simulink model "R19_Modelo_control_CORRIENTE_c_2GDL_2021"  (R2019a)
settings: Solver=ode45  StartTime=0.0  StopTime=20  RelTol=1e-9
undefined symbols (not defined in the file): currentSensorNoise, DiscIntNeverNeededParam, dtCurrent, dTSensor, filterConstant, initial_conds, K_c, Ki, Kp, Lcoil, noiseSensor, pod, Rcoil, T, tauFilterCurrent, z_0, z_ini
libraries: simulink x3, shared3dof x1, cstblocks x1, simulink_extras x1
settings Model: Creator=skapa  LastModifiedBy=emate
settings DataIOCC: LimitDataPoints=on  SaveFormat=Array  SignalLoggingSaveFormat=ModelDataLogs  ReturnWorkspaceOutputs=off
settings OptimizationCC: BlockReduction=off  BooleanDataType=off  LifeSpan=inf
settings DebuggingCC: SaveWithParameterizedLinksMsg=none  UnderspecifiedInitializationDetection=Classic  MergeDetectMultiDrivingBlocksExec=none  SignalResolutionControl=TryResolveAllWithWarning  MultiTaskDSMMsg=warning  MultiTaskCondExecSysMsg=none  SFUnexpectedBacktrackingDiag=warning  SFNoUnconditionalDefaultTransitionDiag=warning  SFExecutionAtInitializationDiag=none  ArithmeticOperatorsInVariantConditions=warning
settings HardwareCC: ProdBitPerPointer=32  ProdBitPerSizeT=32  ProdBitPerPtrDiffT=32  ProdLargestAtomicFloat=None  ProdIntDivRoundTo=Undefined  ProdEndianess=Unspecified  ProdWordSize=32  ProdHWDeviceType=32-bit Generic  TargetUnknown=on
settings ModelReferenceCC: PropagateSignalLabelsOutOfModel=off
settings SFSimCC: SimUseLocalCustomCode=off
settings RTWCC: RTWUseLocalCustomCode=off
settings CodeAppCC: StateflowObjectComments=on
settings GRTTargetCC: TargetLangStandard=C89/C90 (ANSI)
settings ConfigComp: CovMetricSettings=dw  CovSaveCumulativeToWorkspaceVar=on  CovSaveSingleToWorkspaceVar=on  CovExternalEMLEnable=off

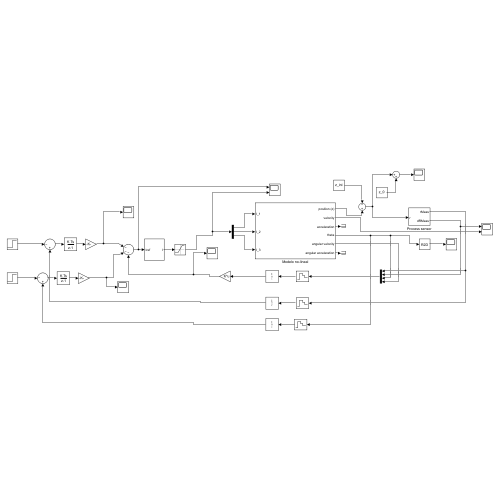
[thumbnail: Simulink's stored preview of the top-level diagram]
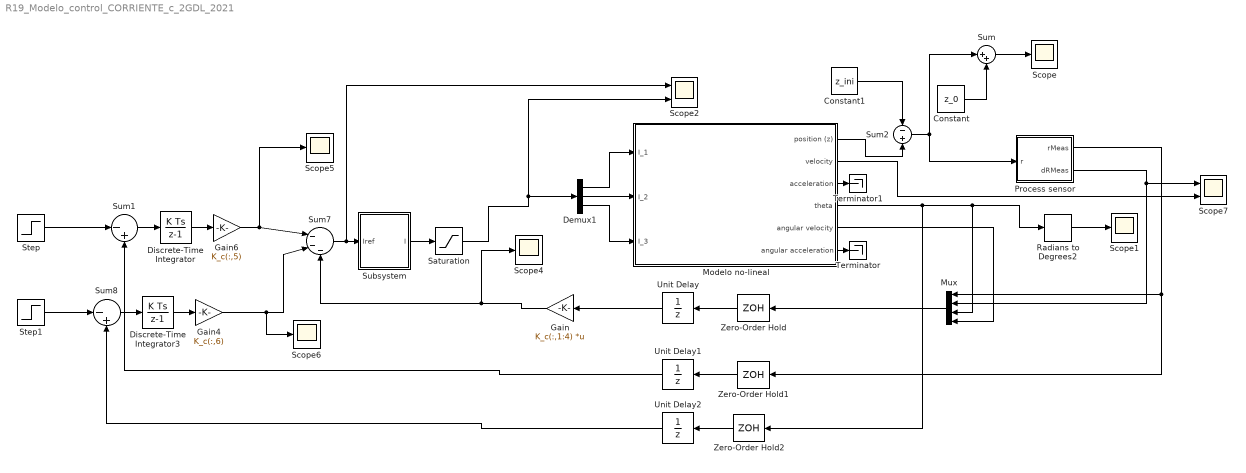
== system R19_Modelo_control_CORRIENTE_c_2GDL_2021 ==
  Constant : Constant  Value=z_0
  Constant1 : Constant  Value=z_ini  SampleTime=T
  Demux1 : Demux  Outputs=3
  Discrete-Time Integrator : DiscreteIntegrator  SampleTime=T  ICPrevOutput=DiscIntNeverNeededParam  ICPrevScaledInput=DiscIntNeverNeededParam
  Discrete-Time Integrator3 : DiscreteIntegrator  SampleTime=T  ICPrevOutput=DiscIntNeverNeededParam  ICPrevScaledInput=DiscIntNeverNeededParam
  Gain : Gain  Gain=K_c(:,1:4)  Multiplication=Matrix(K*u)
  Gain4 : Gain  Gain=K_c(:,6)
  Gain6 : Gain  Gain=K_c(:,5)
  Modelo no-lineal : Subsystem
  Mux : Mux
  Process sensor : Subsystem
  Radians to Degrees2 : simulink_extras/Transformations/Radians to Degrees
  Saturation : Saturate  UpperLimit=40  LowerLimit=-40
  Scope{,1,4..6} (5 alike) : Scope
  Scope2 : Scope  NumInputPorts=2
  Scope7 : Scope  NumInputPorts=2
  Step : Step  Time=0  After=0  SampleTime=T
  Step1 : Step  Time=0  After=0  SampleTime=T
  Subsystem : Subsystem
  Sum : Sum  Inputs=|++
  Sum1 : Sum  Inputs=|-+
  Sum2 : Sum  Inputs=-|+
  Sum7 : Sum  Inputs=|---
  Sum8 : Sum  Inputs=|-+
  Terminator : Terminator
  Terminator1 : Terminator
  Unit Delay : UnitDelay  InitialCondition=[0,0,0,0]  SampleTime=-1  HasFrameUpgradeWarning=on
  Unit Delay1 : UnitDelay  InitialCondition=[0]  SampleTime=-1  HasFrameUpgradeWarning=on
  Unit Delay2 : UnitDelay  InitialCondition=[0]  SampleTime=-1  HasFrameUpgradeWarning=on
  Zero-Order Hold : ZeroOrderHold  SampleTime=T
  Zero-Order Hold1 : ZeroOrderHold  SampleTime=T
  Zero-Order Hold2 : ZeroOrderHold  SampleTime=T
  wires:
  Sum1/1 -> Discrete-Time Integrator/1
  Discrete-Time Integrator/1 -> Gain6/1
  Gain6/1 -> Scope5/1, Sum7/1
  Demux1/1 -> Modelo no-lineal/1(I_1)
  Demux1/2 -> Modelo no-lineal/2(I_2)
  Demux1/3 -> Modelo no-lineal/3(I_3)
  Modelo no-lineal/4(theta) -> Zero-Order Hold2/1, Mux/3, Radians to Degrees2/1
  Modelo no-lineal/6(angular acceleration) -> Terminator/1
  Unit Delay/1 -> Gain/1
  Sum2/1 -> Sum/1, Process sensor/1(r)
  Modelo no-lineal/1(position (z)) -> Sum2/2
  Constant1/1 -> Sum2/1
  Unit Delay1/1 -> Sum1/2
  Step/1 -> Sum1/1
  Gain/1 -> Scope4/1, Sum7/3
  Step1/1 -> Sum8/1
  Discrete-Time Integrator3/1 -> Gain4/1
  Sum8/1 -> Discrete-Time Integrator3/1
  Unit Delay2/1 -> Sum8/2
  Modelo no-lineal/3(acceleration) -> Terminator1/1
  Radians to Degrees2/1 -> Scope1/1
  Saturation/1 -> Scope2/2, Demux1/1
  Zero-Order Hold/1 -> Unit Delay/1
  Zero-Order Hold1/1 -> Unit Delay1/1
  Zero-Order Hold2/1 -> Unit Delay2/1
  Process sensor/1(rMeas) -> Mux/1, Zero-Order Hold1/1
  Modelo no-lineal/5(angular velocity) -> Mux/4
  Mux/1 -> Zero-Order Hold/1
  Process sensor/2(dRMeas) -> Scope7/1, Mux/2
  Modelo no-lineal/2(velocity) -> Scope7/2
  Gain4/1 -> Scope6/1, Sum7/2
  Constant/1 -> Sum/2
  Sum/1 -> Scope/1
  Sum7/1 -> Scope2/1, Subsystem/1(Iref)
  Subsystem/1(I) -> Saturation/1

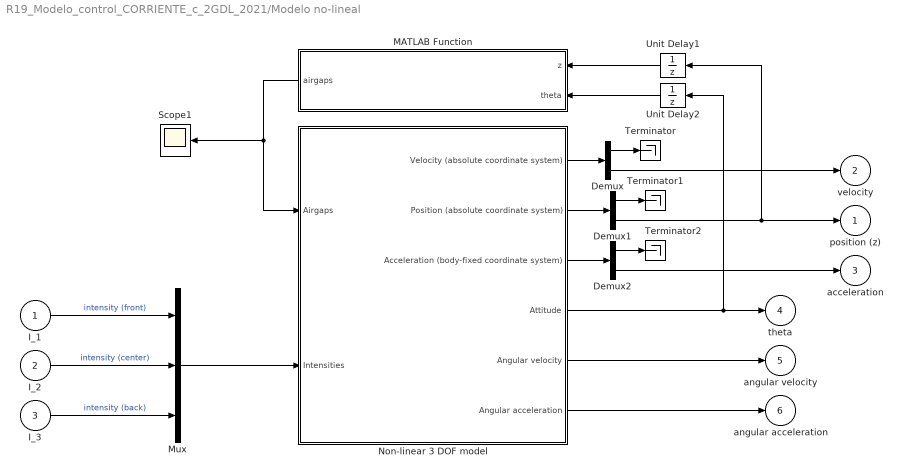
== system R19_Modelo_control_CORRIENTE_c_2GDL_2021/Modelo no-lineal ==
  I_1 : Inport
  I_2 : Inport  Port=2
  I_3 : Inport  Port=3
  Demux : Demux  Outputs=2
  Demux1 : Demux  Outputs=2
  Demux2 : Demux  Outputs=2
  MATLAB Function : MATLAB Function  TreatAsAtomicUnit=on
  Mux : Mux  Inputs=3
  Non-linear 3 DOF model : Subsystem  AncestorBlock=libH7_3DOF/Non-linear 3 DOF model
  Scope1 : Scope
  Terminator : Terminator
  Terminator1 : Terminator
  Terminator2 : Terminator
  Unit Delay1 : UnitDelay  InitialCondition=initial_conds.x_0(3)  SampleTime=-1  HasFrameUpgradeWarning=on
  Unit Delay2 : UnitDelay  SampleTime=-1  HasFrameUpgradeWarning=on
  position (z) : Outport
  velocity : Outport  Port=2
  acceleration : Outport  Port=3
  theta : Outport  Port=4
  angular velocity : Outport  Port=5
  angular acceleration : Outport  Port=6
  wires:
  Mux/1 -> Non-linear 3 DOF model/2(Intensities)
  I_1/1 -> Mux/1  "intensity (front)"
  I_2/1 -> Mux/2  "intensity (center)"
  I_3/1 -> Mux/3  "intensity (back)"
  Non-linear 3 DOF model/4("Attitude ") -> theta/1, Unit Delay2/1
  Non-linear 3 DOF model/5(Angular velocity) -> angular velocity/1
  Non-linear 3 DOF model/1(Velocity (absolute coordinate system)) -> Demux/1
  Demux/1 -> Terminator/1
  Demux/2 -> velocity/1
  Demux1/1 -> Terminator1/1
  Demux1/2 -> Unit Delay1/1, position (z)/1
  Non-linear 3 DOF model/2(Position (absolute coordinate system)) -> Demux1/1
  Demux2/1 -> Terminator2/1
  Demux2/2 -> acceleration/1
  Non-linear 3 DOF model/3(Acceleration (body-fixed coordinate system)) -> Demux2/1
  Unit Delay1/1 -> MATLAB Function/1(z)
  Unit Delay2/1 -> MATLAB Function/2(theta)
  MATLAB Function/1(airgaps) -> Scope1/1, Non-linear 3 DOF model/1(Airgaps)
  Non-linear 3 DOF model/6(Angular acceleration) -> angular acceleration/1

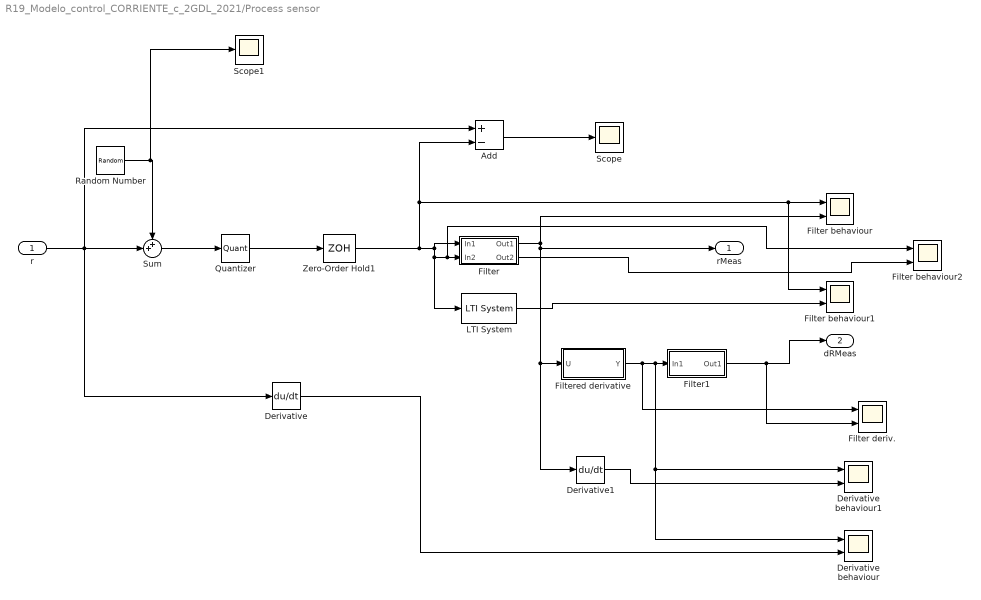
== system R19_Modelo_control_CORRIENTE_c_2GDL_2021/Process sensor ==
  r : Inport
  Add : Sum  Inputs=+-
  Derivative : Derivative
  Derivative behaviour : Scope  NumInputPorts=2
  Derivative behaviour1 : Scope  NumInputPorts=2
  Derivative1 : Derivative
  Filter : Subsystem
  Filter behaviour : Scope  NumInputPorts=2
  Filter behaviour1 : Scope  NumInputPorts=2
  Filter behaviour2 : Scope  NumInputPorts=2
  Filter deriv. : Scope  NumInputPorts=2
  Filter1 : Subsystem
  Filtered derivative : Subsystem
  LTI System : cstblocks/LTI System  sys=Fd_1  IC=[]
  Quantizer : Quantizer  QuantizationInterval=resSensor
  Random Number : RandomNumber  Variance=noiseSensor^2
  Scope : Scope
  Scope1 : Scope
  Sum : Sum  Inputs=++|
  Zero-Order Hold1 : ZeroOrderHold  SampleTime=dTSensor
  rMeas : Outport
  dRMeas : Outport  Port=2
  wires:
  r/1 -> Add/1, Sum/2, Derivative/1
  Random Number/1 -> Sum/1, Scope1/1
  Sum/1 -> Quantizer/1
  Quantizer/1 -> Zero-Order Hold1/1
  Add/1 -> Scope/1
  Zero-Order Hold1/1 -> Add/2, Filter behaviour/1, Filter behaviour1/1, LTI System/1, Filter behaviour2/1, Filter/2(In2), Filter/1(In1)
  Filter/1(Out1) -> Derivative1/1, Filtered derivative/1(U), rMeas/1, Filter behaviour/2
  Derivative/1 -> Derivative behaviour/2
  LTI System/1 -> Filter behaviour1/2
  Filtered derivative/1(Y) -> Filter deriv./1, Filter1/1(In1), Derivative behaviour/1, Derivative behaviour1/1
  Derivative1/1 -> Derivative behaviour1/2
  Filter1/1(Out1) -> Filter deriv./2, dRMeas/1
  Filter/2(Out2) -> Filter behaviour2/2

== system R19_Modelo_control_CORRIENTE_c_2GDL_2021/Subsystem ==
  Iref : Inport
  Closed loop Coil : Subsystem
  Closed loop Coil1 : Subsystem
  Closed loop Coil2 : Subsystem
  Demux : Demux  Outputs=3
  Mux : Mux  Inputs=3
  Zero-Order Hold : ZeroOrderHold  SampleTime=dtCurrent
  I : Outport
  wires:
  Iref/1 -> Zero-Order Hold/1
  Demux/1 -> Closed loop Coil/1(Iref)
  Demux/2 -> Closed loop Coil1/1(Iref)
  Demux/3 -> Closed loop Coil2/1(Iref)
  Closed loop Coil/1(I) -> Mux/1
  Closed loop Coil1/1(I) -> Mux/2
  Closed loop Coil2/1(I) -> Mux/3
  Mux/1 -> I/1
  Zero-Order Hold/1 -> Demux/1

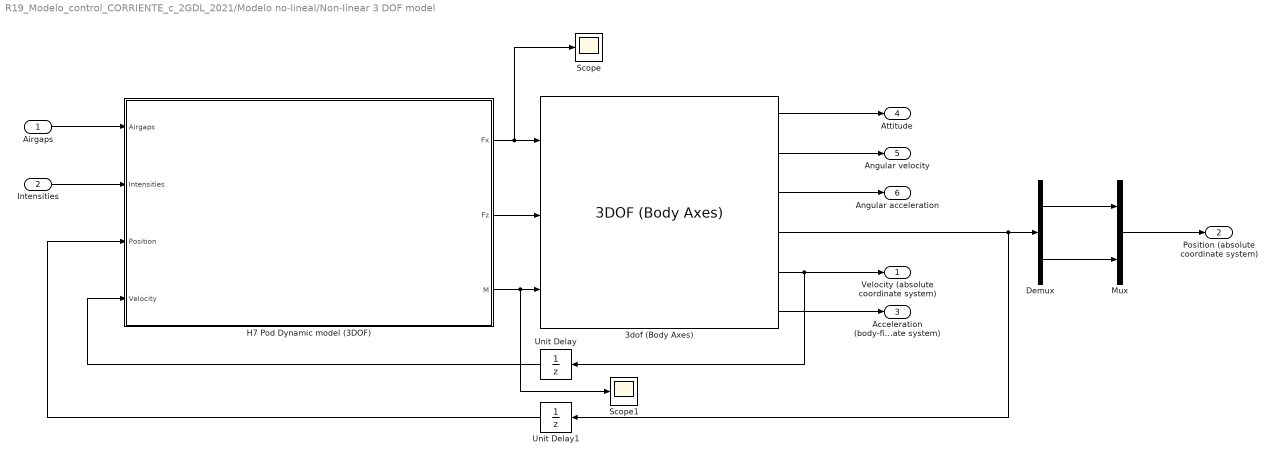
== system R19_Modelo_control_CORRIENTE_c_2GDL_2021/Modelo no-lineal/Non-linear 3 DOF model ==
  Airgaps : Inport
  Intensities : Inport  Port=2
  3dof (Body Axes) : shared3dof/3DOF (Body Axes)  units=Metric (MKS)  mtype=Fixed  v_ini=1e-10  theta_ini=initial_conds.ang_0(2)  alpha_ini=0  pos_ini=initial_conds.x_0(1:2:3)  q_ini=initial_conds.w_0(2)  mass=pod.mass.mass  mass_e=0.5  mass_f=3.0  Iyy=pod.mass.inertia(2,2)  Iyy_e=0.5  Iyy_f=3.0  g_in=Internal  g=9.81  vre_flag=off  abi_flag=off  aMode=0  vel_statename=''  theta_statename=''  pos_statename=''  q_statename=''  mass_statename=''
      settings: SourceProductBaseCode=AE,PW,DR,MT,UV,VE
  Demux : Demux  Outputs=2
  H7 Pod Dynamic model (3DOF) : Subsystem  AncestorBlock=libH7_3DOF/H7 Pod Dynamic model (3DOF)
      mask Display: image('FBD_2D.png', [0.12 0.12 0.78 0.78]); % Use "Edit Image" on toolstrip to change.
  Mux : Mux  Inputs=2
  Scope : Scope
  Scope1 : Scope
  Unit Delay : UnitDelay  InitialCondition=[0,0]  SampleTime=-1  HasFrameUpgradeWarning=on
  Unit Delay1 : UnitDelay  InitialCondition=initial_conds.x_0(1:2:3)  SampleTime=-1  HasFrameUpgradeWarning=on
  Velocity (absolute coordinate system) : Outport
  Position (absolute coordinate system) : Outport  Port=2
  Acceleration (body-fixed coordinate system) : Outport  Port=3
  "Attitude " : Outport  Port=4
  Angular velocity : Outport  Port=5
  Angular acceleration : Outport  Port=6
  wires:
  Demux/2 -> Mux/2
  Demux/1 -> Mux/1
  Unit Delay1/1 -> H7 Pod Dynamic model (3DOF)/3(Position)
  Unit Delay/1 -> H7 Pod Dynamic model (3DOF)/4(Velocity)
  Mux/1 -> Position (absolute coordinate system)/1
  3dof (Body Axes)/1 -> "Attitude "/1
  3dof (Body Axes)/4 -> Unit Delay1/1, Demux/1
  3dof (Body Axes)/5 -> Unit Delay/1, Velocity (absolute coordinate system)/1
  3dof (Body Axes)/3 -> Angular acceleration/1
  3dof (Body Axes)/6 -> Acceleration (body-fixed coordinate system)/1
  Airgaps/1 -> H7 Pod Dynamic model (3DOF)/1(Airgaps)
  Intensities/1 -> H7 Pod Dynamic model (3DOF)/2(Intensities)
  H7 Pod Dynamic model (3DOF)/2(Fz) -> 3dof (Body Axes)/2
  H7 Pod Dynamic model (3DOF)/3(M) -> Scope1/1, 3dof (Body Axes)/3
  3dof (Body Axes)/2 -> Angular velocity/1
  H7 Pod Dynamic model (3DOF)/1(Fx) -> Scope/1, 3dof (Body Axes)/1

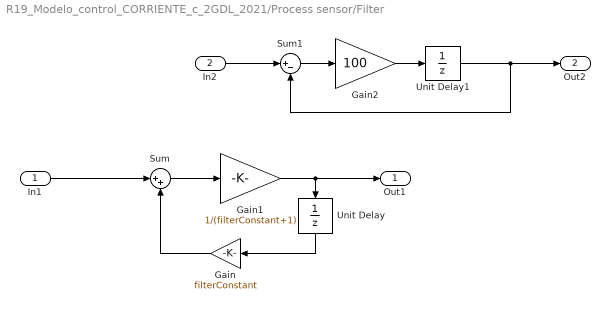
== system R19_Modelo_control_CORRIENTE_c_2GDL_2021/Process sensor/Filter ==
  In1 : Inport
  In2 : Inport  Port=2
  Gain : Gain  Gain=filterConstant
  Gain1 : Gain  Gain=1/(filterConstant+1)
  Gain2 : Gain  Gain=100
  Sum : Sum  Inputs=|++
  Sum1 : Sum  Inputs=|+-
  Unit Delay : UnitDelay  SampleTime=dTSensor  HasFrameUpgradeWarning=on
  Unit Delay1 : UnitDelay  SampleTime=dTSensor  HasFrameUpgradeWarning=on
  Out1 : Outport
  Out2 : Outport  Port=2
  wires:
  In1/1 -> Sum/1
  Gain/1 -> Sum/2
  Sum/1 -> Gain1/1
  Gain1/1 -> Unit Delay/1, Out1/1
  Unit Delay/1 -> Gain/1
  In2/1 -> Sum1/1
  Unit Delay1/1 -> Sum1/2, Out2/1
  Sum1/1 -> Gain2/1
  Gain2/1 -> Unit Delay1/1

== system R19_Modelo_control_CORRIENTE_c_2GDL_2021/Process sensor/Filter1 ==
  In1 : Inport
  Gain : Gain  Gain=10
  Gain1 : Gain  Gain=1/(10+1)
  Sum : Sum  Inputs=|++
  Unit Delay : UnitDelay  SampleTime=dTSensor  HasFrameUpgradeWarning=on
  Out1 : Outport
  wires:
  Unit Delay/1 -> Gain/1
  Gain1/1 -> Out1/1, Unit Delay/1
  Sum/1 -> Gain1/1
  Gain/1 -> Sum/2
  In1/1 -> Sum/1

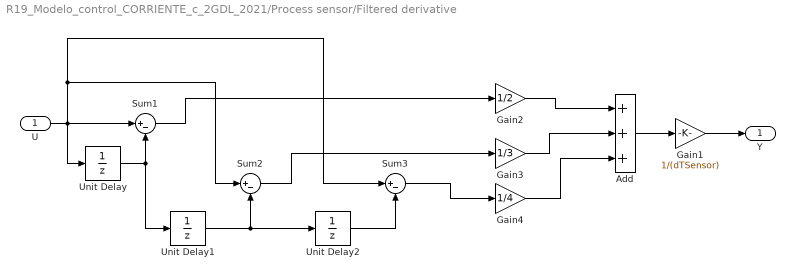
== system R19_Modelo_control_CORRIENTE_c_2GDL_2021/Process sensor/Filtered derivative ==
  U : Inport
  Add : Sum  Inputs=+++
  Gain1 : Gain  Gain=1/(dTSensor)
  Gain2 : Gain  Gain=1/2
  Gain3 : Gain  Gain=1/3
  Gain4 : Gain  Gain=1/4
  Sum1 : Sum  Inputs=|+-
  Sum2 : Sum  Inputs=|+-
  Sum3 : Sum  Inputs=|+-
  Unit Delay : UnitDelay  SampleTime=dTSensor  HasFrameUpgradeWarning=on
  Unit Delay1 : UnitDelay  SampleTime=dTSensor  HasFrameUpgradeWarning=on
  Unit Delay2 : UnitDelay  SampleTime=dTSensor  HasFrameUpgradeWarning=on
  Y : Outport
  wires:
  U/1 -> Sum1/1, Sum2/1, Sum3/1, Unit Delay/1
  Unit Delay/1 -> Sum1/2, Unit Delay1/1
  Unit Delay2/1 -> Sum3/2
  Unit Delay1/1 -> Unit Delay2/1, Sum2/2
  Add/1 -> Gain1/1
  Gain1/1 -> Y/1
  Gain4/1 -> Add/3
  Gain3/1 -> Add/2
  Gain2/1 -> Add/1
  Sum1/1 -> Gain2/1
  Sum2/1 -> Gain3/1
  Sum3/1 -> Gain4/1

== system R19_Modelo_control_CORRIENTE_c_2GDL_2021/Subsystem/Closed loop Coil ==
  Iref : Inport
  Controller : Subsystem
  Open Loop : Subsystem
  Sensor : Subsystem
  Sum : Sum  Inputs=|+-
  I : Outport
  wires:
  Controller/1(V) -> Open Loop/1(V)
  Open Loop/1(I) -> Sensor/1(Ireal), I/1
  Iref/1 -> Sum/1
  Sum/1 -> Controller/1(Iref)
  Sensor/1(Icontrol) -> Sum/2

== system R19_Modelo_control_CORRIENTE_c_2GDL_2021/Subsystem/Closed loop Coil1 ==
  Iref : Inport
  Controller : Subsystem
  Open Loop : Subsystem
  Scope : Scope
  Sensor : Subsystem
  Sum : Sum  Inputs=|+-
  I : Outport
  wires:
  Sensor/1(Icontrol) -> Sum/2
  Sum/1 -> Controller/1(Iref)
  Iref/1 -> Sum/1
  Open Loop/1(I) -> I/1, Sensor/1(Ireal)
  Controller/1(V) -> Open Loop/1(V), Scope/1

== system R19_Modelo_control_CORRIENTE_c_2GDL_2021/Subsystem/Closed loop Coil2 ==
  Iref : Inport
  Controller : Subsystem
  Open Loop : Subsystem
  Scope : Scope
  Sensor : Subsystem
  Sum : Sum  Inputs=|+-
  I : Outport
  wires:
  Controller/1(V) -> Scope/1, Open Loop/1(V)
  Open Loop/1(I) -> Sensor/1(Ireal), I/1
  Iref/1 -> Sum/1
  Sum/1 -> Controller/1(Iref)
  Sensor/1(Icontrol) -> Sum/2

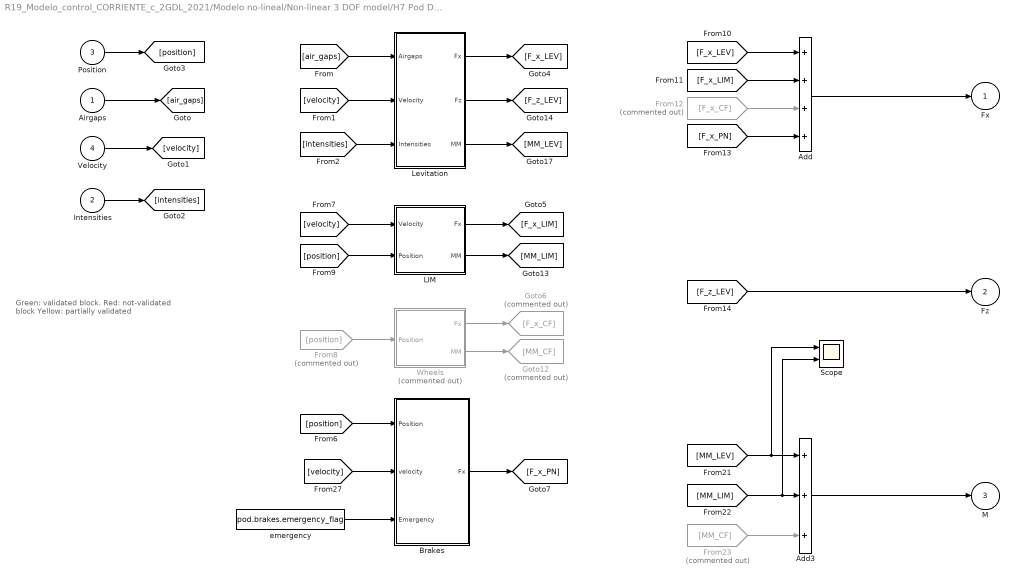
== system R19_Modelo_control_CORRIENTE_c_2GDL_2021/Modelo no-lineal/Non-linear 3 DOF model/H7 Pod Dynamic model (3DOF) ==
  note: Green: validated block.
      | Red: not-validated block
      | Yellow: partially validated
  Airgaps : Inport
  Intensities : Inport  Port=2
  Position : Inport  Port=3
  Velocity : Inport  Port=4
  Add : Sum  Inputs=++++
  Add3 : Sum  Inputs=+++
  "Brakes " : Subsystem  AncestorBlock=libH7/H7 Pod Dynamic model/Brakes
  From12 : From  Commented=on  GotoTag=F_x_CF
  From23 : From  Commented=on  GotoTag=MM_CF
  From8 : From  Commented=on  GotoTag=position
  Goto12 : Goto  Commented=on  GotoTag=MM_CF
  Goto6 : Goto  Commented=on  GotoTag=F_x_CF
  "LIM " : Subsystem  AncestorBlock=libH7/H7 Pod Dynamic model/LIM
  "Levitation " : Subsystem  AncestorBlock=libH7/H7 Pod Dynamic model/Levitation
  Scope : Scope  NumInputPorts=2
  "Wheels " : Subsystem  Commented=on  AncestorBlock=libH7/H7 Pod Dynamic model/Wheels
  emergency : Constant  Value=pod.brakes.emergency_flag
  Fx : Outport
  Fz : Outport  Port=2
  M : Outport  Port=3
  wires:
  "Levitation "/2(Fz) -> [F_z_LEV]
  emergency/1 -> "Brakes "/3(Emergency)
  "LIM "/1(Fx) -> [F_x_LIM]
  [air_gaps] -> "Levitation "/1(Airgaps)
  "Levitation "/1(Fx) -> [F_x_LEV]
  From12/1 -> Add/3
  "LIM "/2(MM) -> [MM_LIM]
  [position] -> "LIM "/2(Position)
  "Levitation "/3(MM) -> [MM_LEV]
  [MM_LEV] -> Scope/1, Add3/1
  [F_z_LEV] -> Fz/1
  [F_x_LEV] -> Add/1
  Intensities/1 -> [intensities]
  [F_x_PN] -> Add/4
  "Brakes "/1(Fx) -> [F_x_PN]
  [F_x_LIM] -> Add/2
  Add/1 -> Fx/1
  From23/1 -> Add3/3
  From8/1 -> "Wheels "/1(Position)
  Airgaps/1 -> [air_gaps]
  Position/1 -> [position]
  [velocity] -> "Levitation "/2(Velocity)
  Add3/1 -> M/1
  Velocity/1 -> [velocity]
  [velocity] -> "Brakes "/2(velocity)
  [MM_LIM] -> Scope/2, Add3/2
  [intensities] -> "Levitation "/3(Intensities)
  [position] -> "Brakes "/1(Position)
  [velocity] -> "LIM "/1(Velocity)
  "Wheels "/1(Fx) -> Goto6/1
  "Wheels "/2(MM) -> Goto12/1

== system R19_Modelo_control_CORRIENTE_c_2GDL_2021/Subsystem/Closed loop Coil/Controller ==
  Iref : Inport
  PID Controller : simulink/Continuous/PID Controller  Controller=PID  Form=Parallel  TimeDomain=Discrete-time  SampleTime=dtCurrent  IntegratorMethod=Forward Euler  ControllerParametersSource=internal  P=Kp  I=Ki  D=0  UseFilter=on  N=100  TunerSelectOption=Transfer Function Based (PID Tuner App)  InitialConditionSource=internal  InitialConditionForIntegrator=0  InitialConditionForFilter=0  DifferentiatorICPrevScaledInput=0  ExternalReset=none  TrackingMode=off  Kt=1  LimitOutput=on  UpperSaturationLimit=48  LowerSaturationLimit=-48  LinearizeAsGain=on  AntiWindupMode=clamping  Kb=1  POutMin=[]  POutMax=[]  IOutMin=[]  IOutMax=[]  DOutMin=[]  DOutMax=[]  NOutMin=[]  NOutMax=[]  SumOutMin=[]  SumOutMax=[]  SaturationOutMin=[]  SaturationOutMax=[]  PParamMin=[]  PParamMax=[]  IParamMin=[]  IParamMax=[]  DParamMin=[]  DParamMax=[]  NParamMin=[]  NParamMax=[]  KbParamMin=[]  KbParamMax=[]  KtParamMin=[]  KtParamMax=[]  KbOutMin=[]  KbOutMax=[]  KtOutMin=[]  KtOutMax=[]  IntegratorOutMin=[]  IntegratorOutMax=[]  FilterOutMin=[]  FilterOutMax=[]  SumI1OutMin=[]  SumI1OutMax=[]  SumI2OutMin=[]  SumI2OutMax=[]  SumI3OutMin=[]  SumI3OutMax=[]  SumI4OutMin=[]  SumI4OutMax=[]  SumDOutMin=[]  SumDOutMax=[]  DifferentiatorOutMin=[]  DifferentiatorOutMax=[]  FilterDiffOutCoefMin=[]  FilterDiffOutCoefMax=[]  ReciprocalOutMin=[]  ReciprocalOutMax=[]  SumDenOutMin=[]  SumDenOutMax=[]  SumNumOutMin=[]  SumNumOutMax=[]  DivideOutMin=[]  DivideOutMax=[]  IntegratorContinuousStateAttributes=''  IntegratorStateMustResolveToSignalObject=off  IntegratorRTWStateStorageClass=Auto  FilterContinuousStateAttributes=''  FilterStateMustResolveToSignalObject=off  FilterRTWStateStorageClass=Auto  ParallelPVariant=InternalParameters  IdealPVariant=Disabled  IVariant=InternalParameters  DVariant=InternalParameters  IntegratorVariant=Discrete  SatVariant=Enabled  AWVariant=DiscClampingParallel  PCopyVariant=Disabled  TRVariant=Disabled  FdbkBlocksVariant=Forward  IdealPFdbkVariant=Disabled  SatFdbkVariant=Disabled  DerivativeFilterVariant=ForwardEulerFilter  NVariant=InternalParameters  NCopyVariant=Disabled  FilterICVariant=InternalICsFilter  IntegratorICVariant=InternalICs  ExternalResetVariant=Disabled  TRSumVariant=Passthrough  SumFdbkVariant=Disabled  SumVariant=Sum_PID
  Scope : Scope
  V : Outport
  wires:
  PID Controller/1 -> Scope/1, V/1
  Iref/1 -> PID Controller/1

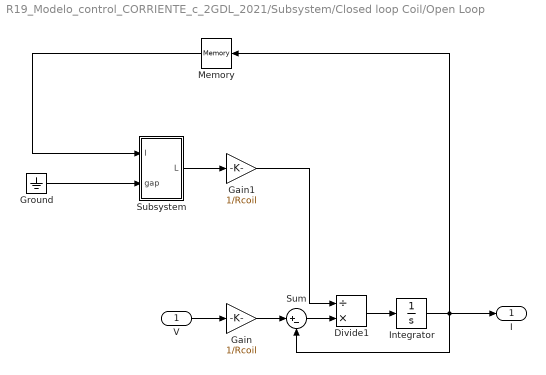
== system R19_Modelo_control_CORRIENTE_c_2GDL_2021/Subsystem/Closed loop Coil/Open Loop ==
  V : Inport
  Divide1 : Product  Inputs=/*
  Gain : Gain  Gain=1/Rcoil
  Gain1 : Gain  Gain=1/Rcoil
  Ground : Ground
  Integrator : Integrator
  Memory : Memory
  Subsystem : Subsystem
  Sum : Sum  Inputs=|+-
  I : Outport
  wires:
  V/1 -> Gain/1
  Gain1/1 -> Divide1/1
  Gain/1 -> Sum/1
  Sum/1 -> Divide1/2
  Divide1/1 -> Integrator/1
  Subsystem/1(L) -> Gain1/1
  Integrator/1 -> Memory/1, Sum/2, I/1
  Memory/1 -> Subsystem/1(I)
  Ground/1 -> Subsystem/2(gap)

== system R19_Modelo_control_CORRIENTE_c_2GDL_2021/Subsystem/Closed loop Coil/Sensor ==
  Ireal : Inport
  Random Number : RandomNumber  Variance=currentSensorNoise  Seed=14
  Scope1 : Scope  NumInputPorts=2
  Sum1 : Sum  Inputs=|++
  Transfer Fcn : TransferFcn  Denominator=[tauFilterCurrent 1]
  Icontrol : Outport
  wires:
  Random Number/1 -> Sum1/2
  Sum1/1 -> Scope1/2, Transfer Fcn/1
  Transfer Fcn/1 -> Icontrol/1, Scope1/1
  Ireal/1 -> Sum1/1

== system R19_Modelo_control_CORRIENTE_c_2GDL_2021/Subsystem/Closed loop Coil1/Controller ==
  Iref : Inport
  PID Controller : simulink/Continuous/PID Controller  Controller=PID  Form=Parallel  TimeDomain=Discrete-time  SampleTime=dtCurrent  IntegratorMethod=Forward Euler  ControllerParametersSource=internal  P=Kp  I=Ki  D=0  UseFilter=on  N=100  TunerSelectOption=Transfer Function Based (PID Tuner App)  InitialConditionSource=internal  InitialConditionForIntegrator=0  InitialConditionForFilter=0  DifferentiatorICPrevScaledInput=0  ExternalReset=none  TrackingMode=off  Kt=1  LimitOutput=on  UpperSaturationLimit=48  LowerSaturationLimit=-48  LinearizeAsGain=on  AntiWindupMode=clamping  Kb=1  POutMin=[]  POutMax=[]  IOutMin=[]  IOutMax=[]  DOutMin=[]  DOutMax=[]  NOutMin=[]  NOutMax=[]  SumOutMin=[]  SumOutMax=[]  SaturationOutMin=[]  SaturationOutMax=[]  PParamMin=[]  PParamMax=[]  IParamMin=[]  IParamMax=[]  DParamMin=[]  DParamMax=[]  NParamMin=[]  NParamMax=[]  KbParamMin=[]  KbParamMax=[]  KtParamMin=[]  KtParamMax=[]  KbOutMin=[]  KbOutMax=[]  KtOutMin=[]  KtOutMax=[]  IntegratorOutMin=[]  IntegratorOutMax=[]  FilterOutMin=[]  FilterOutMax=[]  SumI1OutMin=[]  SumI1OutMax=[]  SumI2OutMin=[]  SumI2OutMax=[]  SumI3OutMin=[]  SumI3OutMax=[]  SumI4OutMin=[]  SumI4OutMax=[]  SumDOutMin=[]  SumDOutMax=[]  DifferentiatorOutMin=[]  DifferentiatorOutMax=[]  FilterDiffOutCoefMin=[]  FilterDiffOutCoefMax=[]  ReciprocalOutMin=[]  ReciprocalOutMax=[]  SumDenOutMin=[]  SumDenOutMax=[]  SumNumOutMin=[]  SumNumOutMax=[]  DivideOutMin=[]  DivideOutMax=[]  IntegratorContinuousStateAttributes=''  IntegratorStateMustResolveToSignalObject=off  IntegratorRTWStateStorageClass=Auto  FilterContinuousStateAttributes=''  FilterStateMustResolveToSignalObject=off  FilterRTWStateStorageClass=Auto  ParallelPVariant=InternalParameters  IdealPVariant=Disabled  IVariant=InternalParameters  DVariant=InternalParameters  IntegratorVariant=Discrete  SatVariant=Enabled  AWVariant=DiscClampingParallel  PCopyVariant=Disabled  TRVariant=Disabled  FdbkBlocksVariant=Forward  IdealPFdbkVariant=Disabled  SatFdbkVariant=Disabled  DerivativeFilterVariant=ForwardEulerFilter  NVariant=InternalParameters  NCopyVariant=Disabled  FilterICVariant=InternalICsFilter  IntegratorICVariant=InternalICs  ExternalResetVariant=Disabled  TRSumVariant=Passthrough  SumFdbkVariant=Disabled  SumVariant=Sum_PID
  V : Outport
  wires:
  Iref/1 -> PID Controller/1
  PID Controller/1 -> V/1

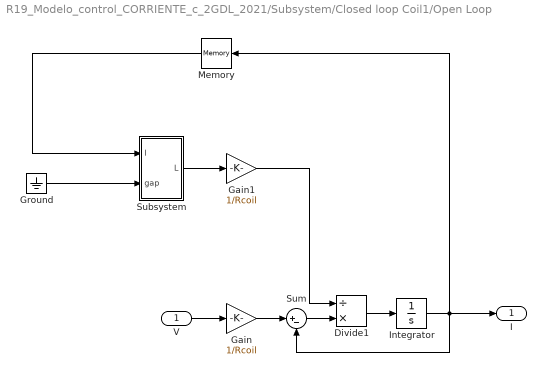
== system R19_Modelo_control_CORRIENTE_c_2GDL_2021/Subsystem/Closed loop Coil1/Open Loop ==
  V : Inport
  Divide1 : Product  Inputs=/*
  Gain : Gain  Gain=1/Rcoil
  Gain1 : Gain  Gain=1/Rcoil
  Ground : Ground
  Integrator : Integrator
  Memory : Memory
  Subsystem : Subsystem
  Sum : Sum  Inputs=|+-
  I : Outport
  wires:
  Ground/1 -> Subsystem/2(gap)
  Memory/1 -> Subsystem/1(I)
  Integrator/1 -> I/1, Sum/2, Memory/1
  Subsystem/1(L) -> Gain1/1
  Divide1/1 -> Integrator/1
  Sum/1 -> Divide1/2
  Gain/1 -> Sum/1
  Gain1/1 -> Divide1/1
  V/1 -> Gain/1

== system R19_Modelo_control_CORRIENTE_c_2GDL_2021/Subsystem/Closed loop Coil1/Sensor ==
  Ireal : Inport
  Random Number : RandomNumber  Variance=currentSensorNoise  Seed=11
  Scope1 : Scope  NumInputPorts=2
  Sum1 : Sum  Inputs=|++
  Transfer Fcn : TransferFcn  Denominator=[tauFilterCurrent 1]
  Icontrol : Outport
  wires:
  Ireal/1 -> Sum1/1
  Transfer Fcn/1 -> Scope1/1, Icontrol/1
  Sum1/1 -> Transfer Fcn/1, Scope1/2
  Random Number/1 -> Sum1/2

== system R19_Modelo_control_CORRIENTE_c_2GDL_2021/Subsystem/Closed loop Coil2/Controller ==
  Iref : Inport
  PID Controller : simulink/Continuous/PID Controller  Controller=PID  Form=Parallel  TimeDomain=Discrete-time  SampleTime=dtCurrent  IntegratorMethod=Forward Euler  ControllerParametersSource=internal  P=Kp  I=Ki  D=0  UseFilter=on  N=100  TunerSelectOption=Transfer Function Based (PID Tuner App)  InitialConditionSource=internal  InitialConditionForIntegrator=0  InitialConditionForFilter=0  DifferentiatorICPrevScaledInput=0  ExternalReset=none  TrackingMode=off  Kt=1  LimitOutput=on  UpperSaturationLimit=48  LowerSaturationLimit=-48  LinearizeAsGain=on  AntiWindupMode=clamping  Kb=1  POutMin=[]  POutMax=[]  IOutMin=[]  IOutMax=[]  DOutMin=[]  DOutMax=[]  NOutMin=[]  NOutMax=[]  SumOutMin=[]  SumOutMax=[]  SaturationOutMin=[]  SaturationOutMax=[]  PParamMin=[]  PParamMax=[]  IParamMin=[]  IParamMax=[]  DParamMin=[]  DParamMax=[]  NParamMin=[]  NParamMax=[]  KbParamMin=[]  KbParamMax=[]  KtParamMin=[]  KtParamMax=[]  KbOutMin=[]  KbOutMax=[]  KtOutMin=[]  KtOutMax=[]  IntegratorOutMin=[]  IntegratorOutMax=[]  FilterOutMin=[]  FilterOutMax=[]  SumI1OutMin=[]  SumI1OutMax=[]  SumI2OutMin=[]  SumI2OutMax=[]  SumI3OutMin=[]  SumI3OutMax=[]  SumI4OutMin=[]  SumI4OutMax=[]  SumDOutMin=[]  SumDOutMax=[]  DifferentiatorOutMin=[]  DifferentiatorOutMax=[]  FilterDiffOutCoefMin=[]  FilterDiffOutCoefMax=[]  ReciprocalOutMin=[]  ReciprocalOutMax=[]  SumDenOutMin=[]  SumDenOutMax=[]  SumNumOutMin=[]  SumNumOutMax=[]  DivideOutMin=[]  DivideOutMax=[]  IntegratorContinuousStateAttributes=''  IntegratorStateMustResolveToSignalObject=off  IntegratorRTWStateStorageClass=Auto  FilterContinuousStateAttributes=''  FilterStateMustResolveToSignalObject=off  FilterRTWStateStorageClass=Auto  ParallelPVariant=InternalParameters  IdealPVariant=Disabled  IVariant=InternalParameters  DVariant=InternalParameters  IntegratorVariant=Discrete  SatVariant=Enabled  AWVariant=DiscClampingParallel  PCopyVariant=Disabled  TRVariant=Disabled  FdbkBlocksVariant=Forward  IdealPFdbkVariant=Disabled  SatFdbkVariant=Disabled  DerivativeFilterVariant=ForwardEulerFilter  NVariant=InternalParameters  NCopyVariant=Disabled  FilterICVariant=InternalICsFilter  IntegratorICVariant=InternalICs  ExternalResetVariant=Disabled  TRSumVariant=Passthrough  SumFdbkVariant=Disabled  SumVariant=Sum_PID
  V : Outport
  wires:
  PID Controller/1 -> V/1
  Iref/1 -> PID Controller/1

== system R19_Modelo_control_CORRIENTE_c_2GDL_2021/Subsystem/Closed loop Coil2/Open Loop ==
  V : Inport
  Divide1 : Product  Inputs=/*
  Gain : Gain  Gain=1/Rcoil
  Gain1 : Gain  Gain=1/Rcoil
  Ground : Ground
  Integrator : Integrator
  Memory : Memory
  Subsystem : Subsystem
  Sum : Sum  Inputs=|+-
  I : Outport
  wires:
  V/1 -> Gain/1
  Gain1/1 -> Divide1/1
  Gain/1 -> Sum/1
  Sum/1 -> Divide1/2
  Divide1/1 -> Integrator/1
  Subsystem/1(L) -> Gain1/1
  Integrator/1 -> Memory/1, Sum/2, I/1
  Memory/1 -> Subsystem/1(I)
  Ground/1 -> Subsystem/2(gap)

== system R19_Modelo_control_CORRIENTE_c_2GDL_2021/Subsystem/Closed loop Coil2/Sensor ==
  Ireal : Inport
  Random Number : RandomNumber  Variance=currentSensorNoise  Seed=7
  Scope1 : Scope  NumInputPorts=2
  Sum1 : Sum  Inputs=|++
  Transfer Fcn : TransferFcn  Denominator=[tauFilterCurrent 1]
  Icontrol : Outport
  wires:
  Random Number/1 -> Sum1/2
  Sum1/1 -> Scope1/1, Transfer Fcn/1
  Transfer Fcn/1 -> Icontrol/1, Scope1/2
  Ireal/1 -> Sum1/1

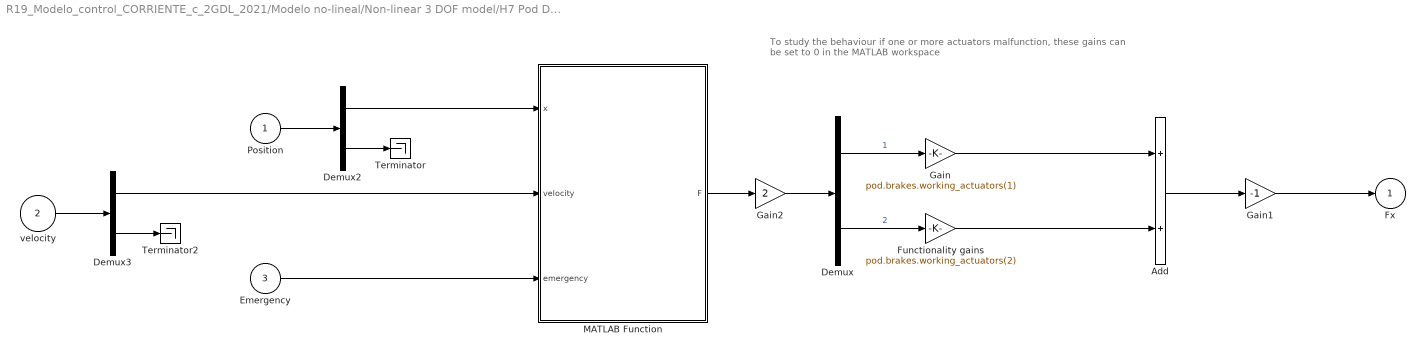
== system R19_Modelo_control_CORRIENTE_c_2GDL_2021/Modelo no-lineal/Non-linear 3 DOF model/H7 Pod Dynamic model (3DOF)/Brakes  ==
  note: To study the behaviour if one or more actuators malfunction,
      | these gains can be set to 0 in the MATLAB workspace
  Position : Inport
  velocity : Inport  Port=2
  Emergency : Inport  Port=3
  Add : Sum
  Demux : Demux  Outputs=2
  Demux2 : Demux  Outputs=2
  Demux3 : Demux  Outputs=2
  Functionality gains : Gain  Gain=pod.brakes.working_actuators(2)
  Gain : Gain  Gain=pod.brakes.working_actuators(1)
  Gain1 : Gain  Gain=-1
  Gain2 : Gain  Gain=2
  MATLAB Function : MATLAB Function  TreatAsAtomicUnit=on
  Terminator : Terminator
  Terminator2 : Terminator
  Fx : Outport
  wires:
  Gain1/1 -> Fx/1
  Add/1 -> Gain1/1
  Gain2/1 -> Demux/1
  Emergency/1 -> MATLAB Function/3(emergency)
  MATLAB Function/1(F) -> Gain2/1
  Demux/1 -> Gain/1  "1"
  Demux/2 -> Functionality gains/1  "2"
  Functionality gains/1 -> Add/2
  Gain/1 -> Add/1
  Position/1 -> Demux2/1
  Demux2/1 -> MATLAB Function/1(x)
  Demux2/2 -> Terminator/1
  velocity/1 -> Demux3/1
  Demux3/2 -> Terminator2/1
  Demux3/1 -> MATLAB Function/2(velocity)

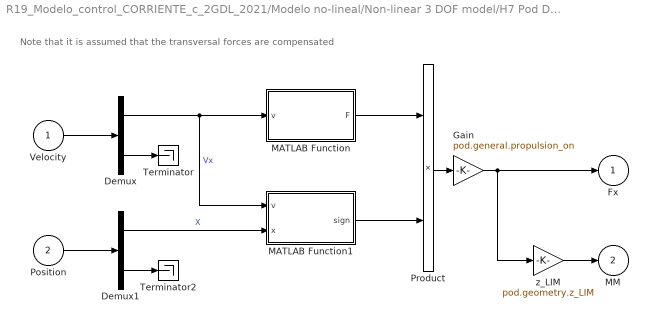
== system R19_Modelo_control_CORRIENTE_c_2GDL_2021/Modelo no-lineal/Non-linear 3 DOF model/H7 Pod Dynamic model (3DOF)/LIM  ==
  note: Note that it is assumed that the transversal forces are compensated
  Velocity : Inport
  Position : Inport  Port=2
  Demux : Demux  Outputs=2
  Demux1 : Demux  Outputs=2
  Gain : Gain  Gain=pod.general.propulsion_on
  MATLAB Function : MATLAB Function  TreatAsAtomicUnit=on
  MATLAB Function1 : MATLAB Function  TreatAsAtomicUnit=on
  Product : Product
  Terminator : Terminator
  Terminator2 : Terminator
  z_LIM : Gain  Gain=pod.geometry.z_LIM
  Fx : Outport
  MM : Outport  Port=2
  wires:
  Gain/1 -> z_LIM/1, Fx/1
  Velocity/1 -> Demux/1
  Demux/2 -> Terminator/1
  Demux/1 -> MATLAB Function/1(v), MATLAB Function1/1(v)  "Vx"
  Position/1 -> Demux1/1
  Demux1/2 -> Terminator2/1
  Demux1/1 -> MATLAB Function1/2(x)  "X"
  MATLAB Function1/1(sign) -> Product/2
  MATLAB Function/1(F) -> Product/1
  Product/1 -> Gain/1
  z_LIM/1 -> MM/1

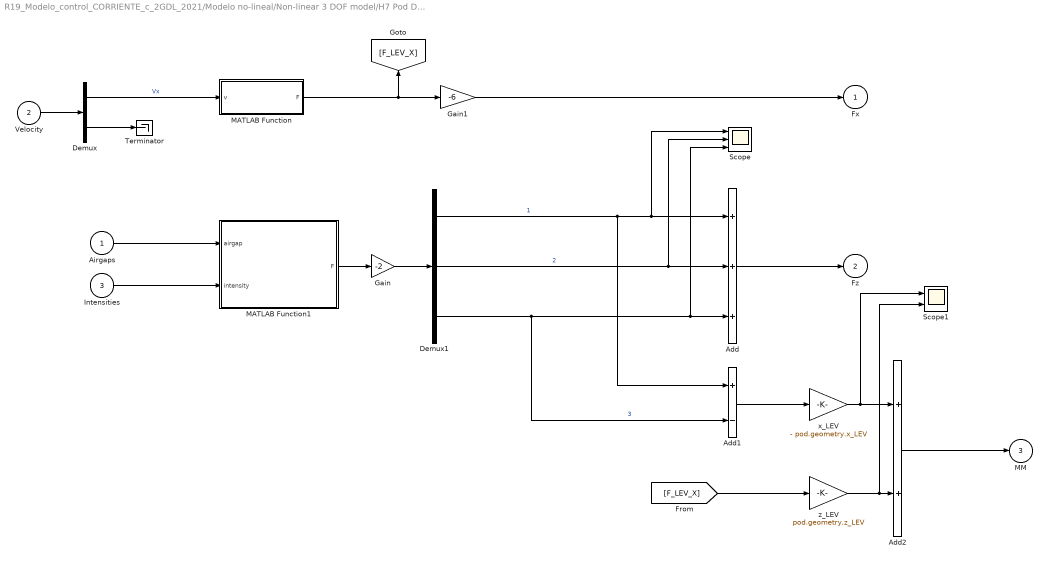
== system R19_Modelo_control_CORRIENTE_c_2GDL_2021/Modelo no-lineal/Non-linear 3 DOF model/H7 Pod Dynamic model (3DOF)/Levitation  ==
  Airgaps : Inport
  Velocity : Inport  Port=2
  Intensities : Inport  Port=3
  Add : Sum  Inputs=+++
  Add1 : Sum  Inputs=+-
  Add2 : Sum
  Demux : Demux  Outputs=2
  Demux1 : Demux  Outputs=3
  Gain : Gain  Gain=-2
  Gain1 : Gain  Gain=-6
  MATLAB Function : MATLAB Function  TreatAsAtomicUnit=on
  MATLAB Function1 : MATLAB Function  TreatAsAtomicUnit=on
  Scope : Scope  NumInputPorts=3
  Scope1 : Scope  NumInputPorts=2
  Terminator : Terminator
  x_LEV : Gain  Gain=- pod.geometry.x_LEV
  z_LEV : Gain  Gain=pod.geometry.z_LEV
  Fx : Outport
  Fz : Outport  Port=2
  MM : Outport  Port=3
  wires:
  Add2/1 -> MM/1
  x_LEV/1 -> Scope1/1, Add2/1
  z_LEV/1 -> Scope1/2, Add2/2
  [F_LEV_X] -> z_LEV/1
  Add1/1 -> x_LEV/1
  Add/1 -> Fz/1
  Demux1/1 -> Scope/1, Add/1, Add1/1  "1"
  Demux1/3 -> Scope/3, Add/3, Add1/2  "3"
  Demux1/2 -> Scope/2, Add/2  "2"
  Gain/1 -> Demux1/1
  Demux/2 -> Terminator/1
  Velocity/1 -> Demux/1
  Demux/1 -> MATLAB Function/1(v)  "Vx"
  Airgaps/1 -> MATLAB Function1/1(airgap)
  Intensities/1 -> MATLAB Function1/2(intensity)
  MATLAB Function1/1(F) -> Gain/1
  MATLAB Function/1(F) -> [F_LEV_X], Gain1/1
  Gain1/1 -> Fx/1

== system R19_Modelo_control_CORRIENTE_c_2GDL_2021/Modelo no-lineal/Non-linear 3 DOF model/H7 Pod Dynamic model (3DOF)/Wheels  ==
  Position : Inport
  Demux : Demux  Outputs=2
  Gain : Gain  Gain=2
  MATLAB Function : MATLAB Function  TreatAsAtomicUnit=on
  Product : Product
  Terminator1 : Terminator
  Fx : Outport
  MM : Outport  Port=2
  wires:
  Gain/1 -> Fx/1, Product/1
  Position/1 -> Demux/1
  Demux/2 -> MATLAB Function/1(z)
  MATLAB Function/1(F) -> Gain/1
  Demux/1 -> Terminator1/1
  MATLAB Function/2(z_CF) -> Product/2
  Product/1 -> MM/1

== system R19_Modelo_control_CORRIENTE_c_2GDL_2021/Subsystem/Closed loop Coil/Open Loop/Subsystem ==
  I : Inport
  gap : Inport  Port=2
  Constant : Constant  Value=Lcoil
  Terminator : Terminator
  Terminator1 : Terminator
  L : Outport
  wires:
  Constant/1 -> L/1
  I/1 -> Terminator/1
  gap/1 -> Terminator1/1

== system R19_Modelo_control_CORRIENTE_c_2GDL_2021/Subsystem/Closed loop Coil1/Open Loop/Subsystem ==
  I : Inport
  gap : Inport  Port=2
  Constant : Constant  Value=Lcoil
  Terminator : Terminator
  Terminator1 : Terminator
  L : Outport
  wires:
  gap/1 -> Terminator1/1
  I/1 -> Terminator/1
  Constant/1 -> L/1

== system R19_Modelo_control_CORRIENTE_c_2GDL_2021/Subsystem/Closed loop Coil2/Open Loop/Subsystem ==
  I : Inport
  gap : Inport  Port=2
  Constant : Constant  Value=Lcoil
  Terminator : Terminator
  Terminator1 : Terminator
  L : Outport
  wires:
  Constant/1 -> L/1
  I/1 -> Terminator/1
  gap/1 -> Terminator1/1

== matlab function R19_Modelo_control_CORRIENTE_c_2GDL_2021/Modelo no-lineal/MATLAB Function ==
  data: z input; theta input; airgaps output; pod parameter
function airgaps = pos2ag2D(z, theta, pod)
% Computes the airgaps (mm) as a function of the position (m) and 
% attitude (rad) of the prototype
% ═════════════════════════════════════════════════════════════════════════
% Last updated: 15.01.2022
% ═════════════════════════════════════════════════════════════════════════

airgaps = zeros(3,1);

airgaps(1) = z - pod.geometry.x_LEV * sin(theta) - pod.geometry.z_LEV * cos(theta);
airgaps(2) = z                                   - pod.geometry.z_LEV * cos(theta);
airgaps(3) = z + pod.geometry.x_LEV * sin(theta) - pod.geometry.z_LEV * cos(theta);

airgaps = airgaps * 1e3;

%if any(airgaps<=11)
%    airgaps = 11 * ones(3,1);
%elseif any(airgaps>=23)
%    airgaps = 23 * ones(3,1);
%end

== matlab function R19_Modelo_control_CORRIENTE_c_2GDL_2021/Modelo no-lineal/Non-linear 3 DOF model/H7 Pod Dynamic model (3DOF)/Brakes /MATLAB Function ==
  data: x input; velocity input; F output; emergency input; pod parameter
function F  = brakes_activation(x, velocity, emergency, pod)
% Computes the braking force of the pneumatic actuators if and only if 
%     (1) The emergency flag has been raised
%     (2) The pod is above the acceleration phase distance
% ═════════════════════════════════════════════════════════════════════════
% Last updated: 20.12.2021
% ═════════════════════════════════════════════════════════════════════════

num_brakes = pod.brakes.n / 2;

if (emergency == 1 && x >= pod.brakes.d && velocity >= 0)
    F       = pod.brakes.force * ones(num_brakes,1);
else
    F       = zeros(num_brakes,1);
end

== matlab function R19_Modelo_control_CORRIENTE_c_2GDL_2021/Modelo no-lineal/Non-linear 3 DOF model/H7 Pod Dynamic model (3DOF)/LIM /MATLAB Function ==
  data: v input; F output; pod parameter
function F = LIMtraction(v, pod)
% Computes the traction force (N) of the LIM as a function of 
% the absolute velocity of the prototype (m/s)
% ═════════════════════════════════════════════════════════════════════════
% Last updated: 20.12.2021
% ═════════════════════════════════════════════════════════════════════════

F = pod.propulsion.poly.p3*v^3 + ...
    pod.propulsion.poly.p2*v^2 + ...
    pod.propulsion.poly.p1*v   + ...
    pod.propulsion.poly.p0;

== matlab function R19_Modelo_control_CORRIENTE_c_2GDL_2021/Modelo no-lineal/Non-linear 3 DOF model/H7 Pod Dynamic model (3DOF)/LIM /MATLAB Function1 ==
  data: v input; x input; sign output; pod parameter
function sign = LIMdirection(v, x, pod)
% Decides if the LIM force is being applied to accelerate or to brake 
% by comparing the position of the pod with a predefined treshold
% ═════════════════════════════════════════════════════════════════════════
% Last updated: 20.12.2021
% ═════════════════════════════════════════════════════════════════════════

if x >= pod.brakes.d && v > 0    
    sign = -1;
elseif x >= pod.brakes.d && v <= 0
    sign = 0;
else
    sign = 1;
end

== matlab function R19_Modelo_control_CORRIENTE_c_2GDL_2021/Modelo no-lineal/Non-linear 3 DOF model/H7 Pod Dynamic model (3DOF)/Levitation /MATLAB Function ==
  data: v input; F output; pod parameter
function F = HEMSdrag(v, pod)
% Computes the drag force (N) of one HEMS unit as a function of the 
% velocity (m/s)
% ═════════════════════════════════════════════════════════════════════════
% Last updated: 16.01.2022
% ═════════════════════════════════════════════════════════════════════════

if v < 1e-3
    v = 0;
end

F = pod.levitation.drag_1_unit.poly.p3*v^3 + ...
    pod.levitation.drag_1_unit.poly.p2*v^2 + ...
    pod.levitation.drag_1_unit.poly.p1*v   + ...
    pod.levitation.drag_1_unit.poly.p0;

== matlab function R19_Modelo_control_CORRIENTE_c_2GDL_2021/Modelo no-lineal/Non-linear 3 DOF model/H7 Pod Dynamic model (3DOF)/Levitation /MATLAB Function1 ==
  data: airgap input; F output; intensity input; pod parameter
function F = HEMSlev(airgap, intensity, pod)
% Computes the levitation force (N) of all the HEMS units as a function of 
% their air gaps (mm) and intensities (A)
% ═════════════════════════════════════════════════════════════════════════
% Last updated: 15.12.2021
% ════════════════════════════════════════════════════════════════════════

x   = airgap;
y   = intensity;

F = pod.levitation.poly_1_unit.p00 + ...
    pod.levitation.poly_1_unit.p10.*x + ...
    pod.levitation.poly_1_unit.p01.*y + ...
    pod.levitation.poly_1_unit.p20.*x.^2 + ...
    pod.levitation.poly_1_unit.p11.*x.*y + ...
    pod.levitation.poly_1_unit.p02.*y.^2 + ...
    pod.levitation.poly_1_unit.p21.*x.^2.*y + ...
    pod.levitation.poly_1_unit.p12.*x.*y.^2 + ...
    pod.levitation.poly_1_unit.p03.*y.^3;

== matlab function R19_Modelo_control_CORRIENTE_c_2GDL_2021/Modelo no-lineal/Non-linear 3 DOF model/H7 Pod Dynamic model (3DOF)/Wheels /MATLAB Function ==
  data: z input; F output; pod parameter; z_CF output
function [F, z_CF] = rollingFriction(z, pod)
% Computes the rolling resistance force (N) of the wheels. It distinguishes
% 3 cases: 
%   (1) z = 0. Pod touching the ground
%   (2) z = z_max. Pod touching the ceiling. It is assumed no current
%   applied to the HEMS. 
%   (3) Otherwise. Pod levitating. 
% ═════════════════════════════════════════════════════════════════════════
% Last updated: 26.12.2021
% ═════════════════════════════════════════════════════════════════════════

% F_LEV worst case scenario computation
x   = 12; % [mm]
y   = 0;  % [A]

F_LEV = pod.levitation.poly_1_unit.p00 + ...
        pod.levitation.poly_1_unit.p10.*x + ...
        pod.levitation.poly_1_unit.p01.*y + ...
        pod.levitation.poly_1_unit.p20.*x.^2 + ...
        pod.levitation.poly_1_unit.p11.*x.*y + ...
        pod.levitation.poly_1_unit.p02.*y.^2 + ...
        pod.levitation.poly_1_unit.p21.*x.^2.*y + ...
        pod.levitation.poly_1_unit.p12.*x.*y.^2 + ...
        pod.levitation.poly_1_unit.p03.*y.^3;

% Main algorithm
if z == 0
    F_N   = pod.mass.mass * 9.81;
    z_CF  = - pod.geometry.z_CF;
elseif z == pod.general.z_range
    F_N   = 6 * F_LEV - pod.mass.mass * 9.81;
    z_CF  = pod.geometry.z_CF;
else
    F_N   = 0;
    z_CF  = 0;
end

F = pod.wheels.number * pod.wheels.roll_coef * F_N;
